simulink model "allActuatorPlant_th"  (R2018b)
settings: Solver=FixedStepAuto  StartTime=0.0  StopTime=duration_s  FixedStep=timeStep_s  RelTol=1e-3
libraries: allActuatorPlant_cl x1
settings Model: Creator=mcobb  LastModifiedBy=mcobb

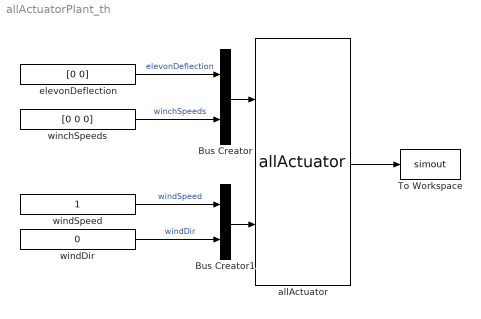
== system allActuatorPlant_th ==
  Bus Creator : BusCreator  Inputs=2  OutDataTypeStr=Bus: ctrlBus
      settings: InheritFromInputs=off
  Bus Creator1 : BusCreator  Inputs=2  OutDataTypeStr=Bus: envBus
  To Workspace : ToWorkspace  VariableName=simout  SaveFormat=Timeseries  SampleTime=-1
  allActuator : allActuatorPlant_cl/allActuator  SystemSampleTime=-1
  elevonDeflection : Constant  Value=[0 0]
  winchSpeeds : Constant  Value=[0 0 0]
  windDir : Constant  Value=0
  windSpeed : Constant
  wires:
  Bus Creator/1 -> allActuator/1
  Bus Creator1/1 -> allActuator/2
  elevonDeflection/1 -> Bus Creator/1  "elevonDeflection"
  winchSpeeds/1 -> Bus Creator/2  "winchSpeeds"
  windDir/1 -> Bus Creator1/2  "windDir"
  windSpeed/1 -> Bus Creator1/1  "windSpeed"
  allActuator/1 -> To Workspace/1
